simulink model "thrust_model"  (R2019b)
settings: Solver=FixedStepAuto  StartTime=0.0  StopTime=10.0  RelTol=1e-3
undefined symbols (not defined in the file): d, hover_T_init, Rn, sim_freq, tau_T, virtual_controls_mat
settings Model: Creator=francois  LastModifiedBy=francois

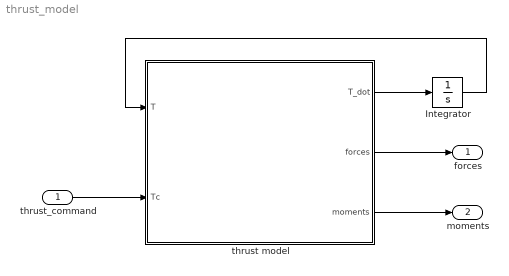
== system thrust_model ==
  thrust_command : Inport  PortDimensions=4
  Integrator : Integrator  InitialCondition=hover_T_init * ones(4,1)
  thrust model : MATLAB Function  TreatAsAtomicUnit=on  SystemSampleTime=1/sim_freq
  forces : Outport
  "moments " : Outport  Port=2
  wires:
  thrust_command/1 -> thrust model/2(Tc)
  thrust model/1(T_dot) -> Integrator/1
  Integrator/1 -> thrust model/1(T)
  thrust model/3(moments) -> "moments "/1
  thrust model/2(forces) -> forces/1

== matlab function thrust_model/thrust model ==
  data: T input; T_dot output; Tc input; forces output; moments output; d parameter; Rn parameter size=1; virtual_controls_mat parameter size=[4,4]; tau_T parameter size=1
function [T_dot, forces, moments] = thrustModel(T, Tc, d, Rn, virtual_controls_mat, tau_T)

T_virtual = virtual_controls_mat*T;
T_dot = (-T + Tc)/tau_T;

forces = [0; 0; -T_virtual(1)];
moments = [d*T_virtual(2); d*T_virtual(3); Rn*T_virtual(4)];

end
